simulink model "Lab01_MotorModel"  (R2019b)
settings: Solver=FixedStepAuto  StartTime=0.0  StopTime=3  FixedStep=0.001  RelTol=1e-3
values from neighbouring files (symbols this model uses):
  b = 0.0088    [DC_Motor_Parameter_Initialization.m]
  J = 0.0021    [DC_Motor_Parameter_Initialization.m]
  Ke = 0.383    [DC_Motor_Parameter_Initialization.m]
  Kt = 0.383    [DC_Motor_Parameter_Initialization.m]
  L = 0.00106    [DC_Motor_Parameter_Initialization.m]
  R = 1.215    [DC_Motor_Parameter_Initialization.m]
settings Model: Creator=Nick  LastModifiedBy=Nick

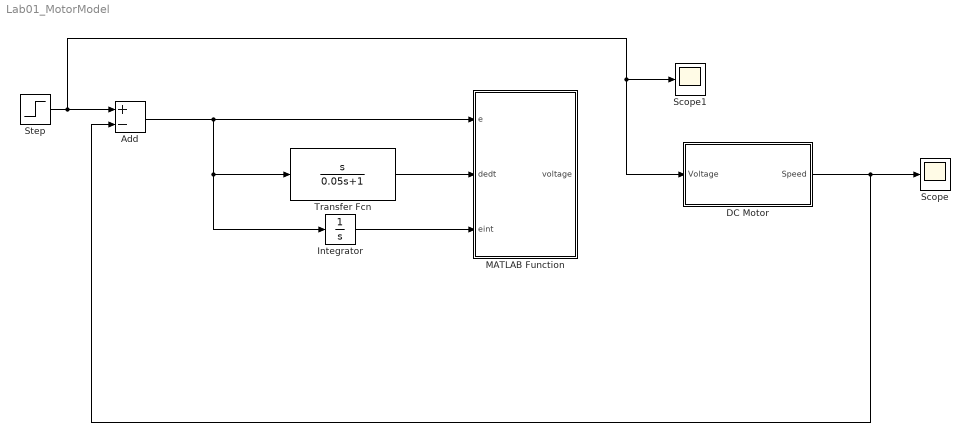
== system Lab01_MotorModel ==
  Add : Sum  Inputs=+-
  DC Motor : Subsystem
  Integrator : Integrator
  MATLAB Function : MATLAB Function  TreatAsAtomicUnit=on
  Scope : Scope
  Scope1 : Scope
  Step : Step  After=12  SampleTime=0
  Transfer Fcn : TransferFcn  Numerator=[1 0]  Denominator=[0.05 1]
  wires:
  Step/1 -> DC Motor/1(Voltage), Scope1/1, Add/1
  DC Motor/1(Speed) -> Add/2, Scope/1
  Add/1 -> Integrator/1, Transfer Fcn/1, MATLAB Function/1(e)
  Transfer Fcn/1 -> MATLAB Function/2(dedt)
  Integrator/1 -> MATLAB Function/3(eint)

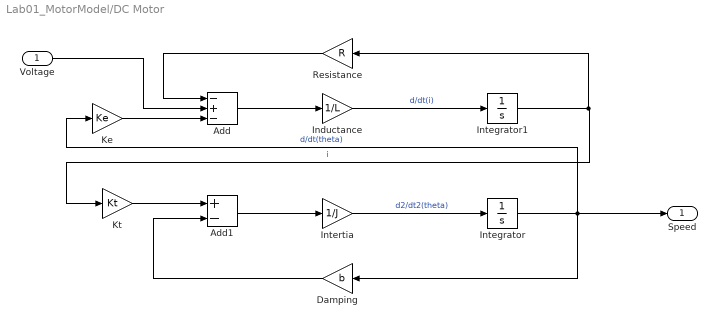
== system Lab01_MotorModel/DC Motor ==
  Voltage : Inport
  Add : Sum  Inputs=-+-
  Add1 : Sum  Inputs=+-
  Damping : Gain  Gain=b
  Inductance : Gain  Gain=1/L
  Integrator : Integrator
  Integrator1 : Integrator
  Intertia : Gain  Gain=1/J
  Ke : Gain  Gain=Ke
  Kt : Gain  Gain=Kt
  Resistance : Gain  Gain=R
  Speed : Outport
  wires:
  Integrator1/1 -> Resistance/1, Kt/1  "i"
  Damping/1 -> Add1/2
  Add/1 -> Inductance/1
  Ke/1 -> Add/3
  Inductance/1 -> Integrator1/1  "d/dt(i)"
  Add1/1 -> Intertia/1
  Voltage/1 -> Add/2
  Integrator/1 -> Speed/1, Ke/1, Damping/1  "d/dt(theta)"
  Resistance/1 -> Add/1
  Kt/1 -> Add1/1
  Intertia/1 -> Integrator/1  "d2/dt2(theta)"

== matlab function Lab01_MotorModel/MATLAB Function ==
  data: e input; voltage output; dedt input; eint input
function voltage = fcn(e, dedt, eint)

Kp = 100;
Ki = 25;
Kd = 10;

minVoltage = 0;
maxVoltage = 12;

voltage = Kp*(e) + Ki*(eint) + Kd*(dedt);

if voltage < minVoltage
    voltage = 0;
elseif voltage > maxVoltage
    voltage = 12;
end
